simulink model "Lab2BlockDiagram"  (R2020a)
settings: Solver=VariableStepAuto  StartTime=0.0  StopTime=4  RelTol=1e-3
values from neighbouring files (symbols this model uses):
  A = [0 1; 0 -1/T]    [Lab2_Code.m]
  B = [0; Kp/T]    [Lab2_Code.m]
  C = [1 0]    [Lab2_Code.m]
  I = eye(2)    [Lab2_Code.m]
  K = [-274.1012 -5.5167]    [Lab2_Code.m]
  L = [62.87; 523.04]    [Lab2_Code.m]
settings Model: Creator=kevin  LastModifiedBy=kevin

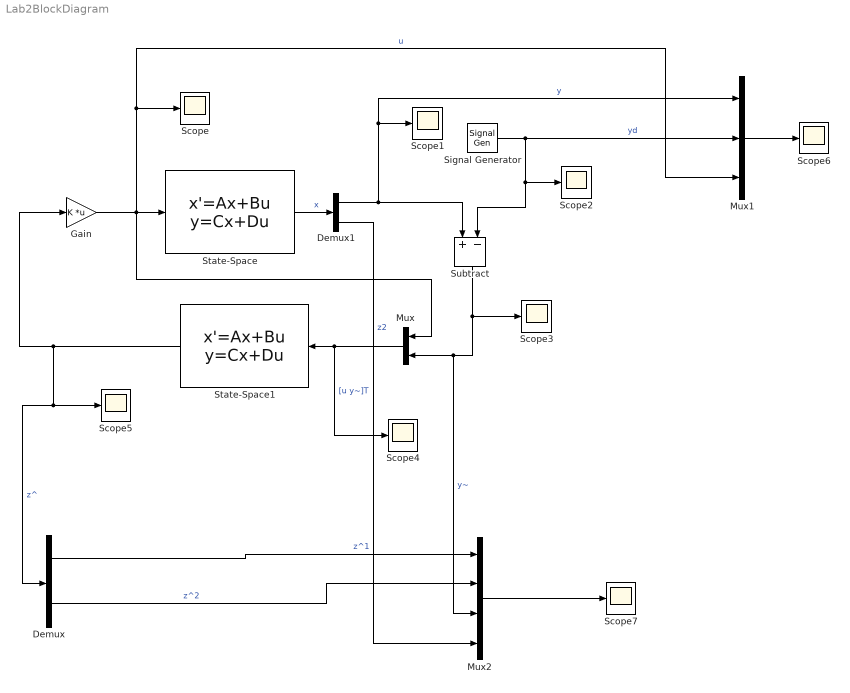
== system Lab2BlockDiagram ==
  Demux : Demux  Outputs=2
  Demux1 : Demux  Outputs=2
  Gain : Gain  Gain=K  Multiplication=Matrix(K*u)
  Mux : Mux  Inputs=2
  Mux1 : Mux  Inputs=3
  Mux2 : Mux
  Scope{,1..7} (8 alike) : Scope
  Signal Generator : SignalGenerator  WaveForm=square  Amplitude=0.015  Frequency=0.5
  State-Space : StateSpace  A=A  B=B  C=[1 0; 0 1]  D=[0 ; 0]  InitialCondition=[0; 0]
  State-Space1 : StateSpace  A=A-L*C  B=[B L]  C=I  D=[0 0; 0 0]  InitialCondition=[0; 0]
  Subtract : Sum  Inputs=+-
  wires:
  State-Space1/1 -> Demux/1, Scope5/1, Gain/1  "z^"
  Subtract/1 -> Scope3/1, Mux2/3, Mux/2  "y~"
  Signal Generator/1 -> Mux1/2, Scope2/1, Subtract/2  "yd"
  Mux/1 -> Scope4/1, State-Space1/1  "[u y~]T"
  Gain/1 -> Scope/1, Mux1/3, Mux/1, State-Space/1  "u"
  Mux2/1 -> Scope7/1
  Mux1/1 -> Scope6/1
  Demux/1 -> Mux2/1  "z^1"
  Demux/2 -> Mux2/2  "z^2"
  State-Space/1 -> Demux1/1  "x"
  Demux1/1 -> Subtract/1, Mux1/1, Scope1/1  "y"
  Demux1/2 -> Mux2/4  "z2"
